simulink model "s6_1"  (R2017a)
settings: Solver=VariableStepAuto  StartTime=0.0  StopTime=0.1  MaxStep=1e-4  RelTol=1e-3
undefined symbols (not defined in the file): m
libraries: powerlib x15, powerlib_meascontrol x1
settings Model: Creator=Lechatelia  LastModifiedBy=Lechatelia

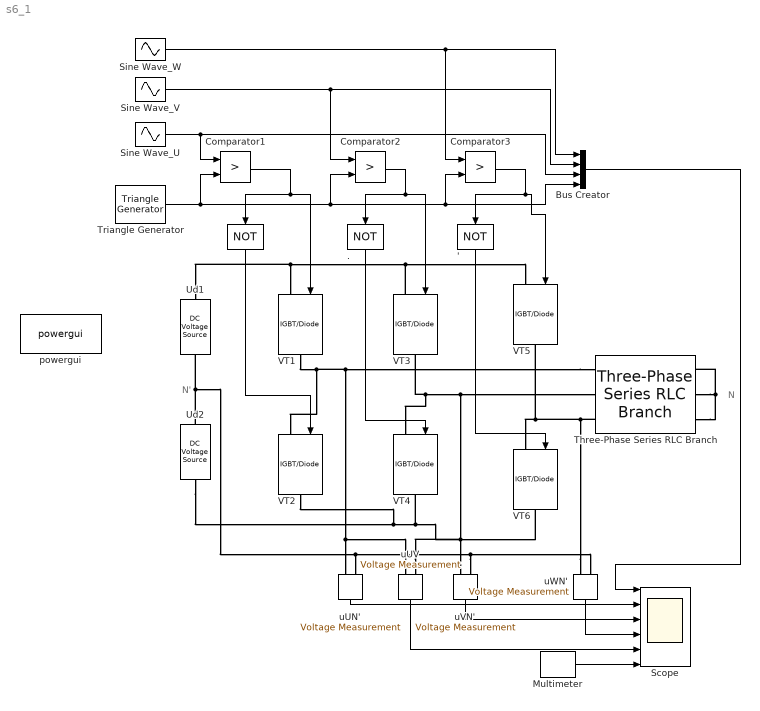
== system s6_1 ==
  note: N
  note: N'
  " " : Logic  Operator=NOT  AllPortsSameDT=off  OutDataTypeStr=boolean
  " '" : Logic  Operator=NOT  AllPortsSameDT=off  OutDataTypeStr=boolean
  " ." : Logic  Operator=NOT  AllPortsSameDT=off  OutDataTypeStr=boolean
  Bus Creator : BusCreator  DialogController=Simulink.DDGSource_Bus  Inputs=4
  Comparator1 : RelationalOperator  Operator=>  OutDataTypeStr=boolean  RndMeth=Nearest
  Comparator2 : RelationalOperator  Operator=>  OutDataTypeStr=boolean  RndMeth=Nearest
  Comparator3 : RelationalOperator  Operator=>  OutDataTypeStr=boolean  RndMeth=Nearest
  Multimeter : powerlib/Measurements/Multimeter  PhasorSimulation=off  OutputType=Complex  sel=1  L=6  Gain=1  yselected={'Ub1: Three-Phase Series RLC Branch'};  PSBOutputType=1  PSBequivalent=0  AxesSetting=[0,0.1,-100,100]  Display=0  SavedBlockNames=-11
  Scope : Scope  NumInputPorts=6
  Sine Wave_U : Sin  Amplitude=m  Frequency=100*pi  SampleTime=0
  Sine Wave_V : Sin  Amplitude=m  Frequency=100*pi  Phase=-2*pi/3  SampleTime=0
  Sine Wave_W : Sin  Amplitude=m  Frequency=100*pi  Phase=2*pi/3  SampleTime=0
  Three-Phase Series RLC Branch : powerlib/Elements/Three-Phase Series RLC Branch  LConnTagsString=A|B|C  RConnTagsString=A|B|C  BranchType=RL  Resistance=10  Inductance=0.004  Capacitance=inf  Measurements=Branch voltages and currents
  Triangle Generator : powerlib_meascontrol/Pulse & Signal Generators/Triangle Generator  Freq=15000  Phase=0  Ts=0
  Ud1 : powerlib/Electrical Sources/DC Voltage Source  Amplitude=425  Measurements=None
  Ud2 : powerlib/Electrical Sources/DC Voltage Source  Amplitude=425  Measurements=None
  VT{1..6} (6 alike) : powerlib/Power Electronics/IGBT//Diode  Ron=0.00  Rs=1e5  Cs=inf  Measurements=off
  powergui : powerlib/powergui  Priority=1  SimulationMode=Continuous  SampleTime=50e-6  frequency=60  Iterations=50  frequencyindice=0  Pbase=100e6  ErrMax=1e-4  UnitsV=kV  UnitsW=MW  buscounter=0  FunctionMessages=off  echomessages=off  EnableUseOfTLC=off  CurrentSourceSwitches=off  DisableSnubberDevices=off  DisableRonSwitches=off  DisableVfSwitches=off  DisplayEquations=off  SolverType=Tustin/Backward Euler (TBE)  Interpol=off  ExternalGateDelay=off  methode=off  Ts=100  x0status=blocks  SPID=on  SwTol=0  HookPort=off  RestoreLinks=warning  ResistiveCurrentMeasurement=off  Frange=[0:2:500]  Ylog=off  Xlog=on  ShowGrid=off  save=off  variable=ZData  structure=ScopeData  ZoomFFT=on  StartTime=0.08  cycles=1  DisplayStyle=1  fundamental=50  FreqAxis=off  MaxFrequency=100000  frequencyindicesteady=1  RmsSteady=1  display=off
  uUN' : powerlib/Measurements/Voltage Measurement  PhasorSimulation=off  OutputType=Complex  PSBequivalent=0
  uUV : powerlib/Measurements/Voltage Measurement  PhasorSimulation=off  OutputType=Complex  PSBequivalent=0
  uVN' : powerlib/Measurements/Voltage Measurement  PhasorSimulation=off  OutputType=Complex  PSBequivalent=0
  uWN' : powerlib/Measurements/Voltage Measurement  PhasorSimulation=off  OutputType=Complex  PSBequivalent=0
  wires:
  " "/1 -> VT2/1
  Bus Creator/1 -> Scope/1
  Sine Wave_V/1 -> Comparator2/1, Bus Creator/2
  " '"/1 -> VT6/1
  uWN'/1 -> Scope/4
  Comparator2/1 -> VT3/1, " ."/1
  Multimeter/1 -> Scope/6
  Comparator1/1 -> VT1/1, " "/1
  " ."/1 -> VT4/1
  Sine Wave_U/1 -> Bus Creator/3, Comparator1/1
  uUV/1 -> Scope/5
  Sine Wave_W/1 -> Comparator3/1, Bus Creator/1
  Comparator3/1 -> VT5/1, " '"/1
  uVN'/1 -> Scope/3
  Triangle Generator/1 -> Comparator1/2, Comparator2/2, Comparator3/2, Bus Creator/4
  uUN'/1 -> Scope/2
  connections:
  Three-Phase Series RLC Branch/RConn1 -- Three-Phase Series RLC Branch/RConn2 -- Three-Phase Series RLC Branch/RConn3
  uVN'/LConn2 -- Ud2/RConn1 -- Ud1/LConn1 -- uUN'/LConn2 -- uWN'/LConn2
  Three-Phase Series RLC Branch/LConn1 -- uUN'/LConn1 -- uUV/LConn1 -- VT2/LConn1 -- VT1/RConn1
  Ud1/RConn1 -- VT1/LConn1 -- VT5/LConn1 -- VT3/LConn1
  Ud2/LConn1 -- VT2/RConn1 -- VT6/RConn1 -- VT4/RConn1
  uUV/LConn2 -- VT4/LConn1 -- VT3/RConn1 -- Three-Phase Series RLC Branch/LConn2 -- uVN'/LConn1
  uWN'/LConn1 -- Three-Phase Series RLC Branch/LConn3 -- VT5/RConn1 -- VT6/LConn1
